simulink model "AssemControl"  (R2013a)
settings: Solver=ode15s  StartTime=0.0  StopTime=13  RelTol=1e-6
values from neighbouring files (symbols this model uses):
  Kd = [0.8784 0.9570 0.8952 0.9813 0.9602 1.0000]*koef*(-1)    [ParametriZaSimulacija.m]
  Ki = [0.1216 0.0430 0.1048 0.0187 0.0398 0]*koef    [ParametriZaSimulacija.m]
  Kp = [1.8784 1.9570 1.8952 1.9813 1.9602 2.0000]*koef*10    [ParametriZaSimulacija.m]
  q_pocetna = q_pocetna*pi/180    [ParametriZaSimulacija.m]
  s = size(xyz)    [PosakuvaniVremetraenja.m]    (also in invkine.m = size(theta_vl))
undefined symbols (not defined in the file or in its folder): X, Y, Z
libraries: sm_lib x450, fl_lib x46, nesl_utility x31
(part 5 of 9)

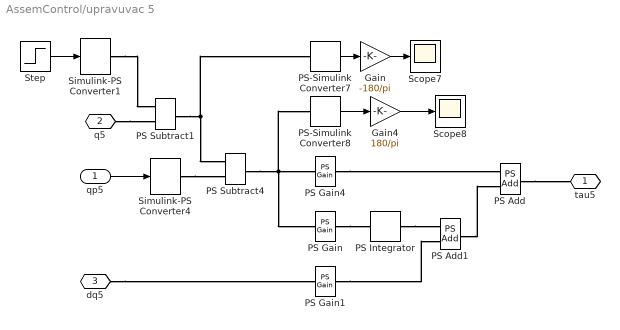
== system AssemControl/upravuvac 5 ==
  qp5 : Inport
  Gain : Gain  Gain=-180/pi
  Gain4 : Gain  Gain=180/pi
  PS Add : fl_lib/Physical Signals/Functions/PS Add  LocalVarLogging=[]
  PS Add1 : fl_lib/Physical Signals/Functions/PS Add  LocalVarLogging=[]
  PS Gain : fl_lib/Physical Signals/Functions/PS Gain  gain=Ki(5)  LocalVarLogging=[]
  PS Gain1 : fl_lib/Physical Signals/Functions/PS Gain  gain=Kd(5)  LocalVarLogging=[]
  PS Gain4 : fl_lib/Physical Signals/Functions/PS Gain  gain=Kp(5)  LocalVarLogging=[]
  PS Integrator : fl_lib/Physical Signals/Linear Operators/PS Integrator  x0=0  x_Log=off  LocalVarNames=|x  LocalVarDescs=|x  LocalVarLogging=0
  PS Subtract1 : fl_lib/Physical Signals/Functions/PS Subtract  LocalVarLogging=[]
  PS Subtract4 : fl_lib/Physical Signals/Functions/PS Subtract  LocalVarLogging=[]
  PS-Simulink Converter7 : nesl_utility/PS-Simulink Converter  PhysicalDomain=network_engine_domain  SubClassName=ps_output  LeftPortType=input  RightPortType=output  PseudoPeriodic=off  Frequencies=[]  Unit=1  AffineConversion=off
  PS-Simulink Converter8 : nesl_utility/PS-Simulink Converter  PhysicalDomain=network_engine_domain  SubClassName=ps_output  LeftPortType=input  RightPortType=output  PseudoPeriodic=off  Frequencies=[]  Unit=1  AffineConversion=off
  Scope7 : Scope
      settings: SaveName=ScopeData14
  Scope8 : Scope
      settings: SaveName=ScopeData3
  Simulink-PS Converter1 : nesl_utility/Simulink-PS Converter  PhysicalDomain=network_engine_domain  SubClassName=ps_input  LeftPortType=input  RightPortType=output  PseudoPeriodic=off  Frequencies=[]  NoiseDistribution=none  NoiseParameters=[]  Unit=1  AffineConversion=off  InputFiltering=off  SimscapeFilterOrder=1  InputFilterTimeConstant=0.001  UdotUserProvided=1
  Simulink-PS Converter4 : nesl_utility/Simulink-PS Converter  PhysicalDomain=network_engine_domain  SubClassName=ps_input  LeftPortType=input  RightPortType=output  PseudoPeriodic=off  Frequencies=[]  NoiseDistribution=none  NoiseParameters=[]  Unit=1  AffineConversion=off  InputFiltering=off  SimscapeFilterOrder=1  InputFilterTimeConstant=0.001  UdotUserProvided=1
  Step : Step  Time=0  Before=q_pocetna(5)  After=q_pocetna(5)  SampleTime=0
  tau5 : PMIOPort  Port=1  Side=Right
  q5 : PMIOPort  Port=2  Side=Left
  dq5 : PMIOPort  Port=3  Side=Left
  wires:
  qp5/1 -> Simulink-PS Converter4/1
  Step/1 -> Simulink-PS Converter1/1
  PS-Simulink Converter8/1 -> Gain4/1
  Gain4/1 -> Scope8/1
  PS-Simulink Converter7/1 -> Gain/1
  Gain/1 -> Scope7/1
  connections:
  PS Subtract1/RConn1 -- PS Subtract4/LConn2 -- PS-Simulink Converter7/LConn1
  PS Subtract4/RConn1 -- PS-Simulink Converter8/LConn1 -- PS Gain4/LConn1 -- PS Gain/LConn1
  Simulink-PS Converter4/RConn1 -- PS Subtract4/LConn1
  PS Add/RConn1 -- tau5/RConn1
  PS Gain4/RConn1 -- PS Add/LConn1
  PS Gain/RConn1 -- PS Integrator/LConn1
  PS Add1/RConn1 -- PS Add/LConn2
  PS Integrator/RConn1 -- PS Add1/LConn1
  PS Gain1/RConn1 -- PS Add1/LConn2
  dq5/RConn1 -- PS Gain1/LConn1
  Simulink-PS Converter1/RConn1 -- PS Subtract1/LConn2
  q5/RConn1 -- PS Subtract1/LConn1

== system AssemControl/upravuvac 6 ==
  qp6 : Inport
  Gain5 : Gain  Gain=-180/pi
  PS Gain5 : fl_lib/Physical Signals/Functions/PS Gain  gain=2000  LocalVarLogging=[]
  PS Subtract1 : fl_lib/Physical Signals/Functions/PS Subtract  LocalVarLogging=[]
  PS Subtract5 : fl_lib/Physical Signals/Functions/PS Subtract  LocalVarLogging=[]
  PS-Simulink Converter5 : nesl_utility/PS-Simulink Converter  PhysicalDomain=network_engine_domain  SubClassName=ps_output  LeftPortType=input  RightPortType=output  PseudoPeriodic=off  Frequencies=[]  Unit=1  AffineConversion=off
  Scope5 : Scope
      settings: YMin=-1.49252  YMax=-1.35038  SaveName=ScopeData11
  Simulink-PS Converter1 : nesl_utility/Simulink-PS Converter  PhysicalDomain=network_engine_domain  SubClassName=ps_input  LeftPortType=input  RightPortType=output  PseudoPeriodic=off  Frequencies=[]  NoiseDistribution=none  NoiseParameters=[]  Unit=1  AffineConversion=off  InputFiltering=off  SimscapeFilterOrder=1  InputFilterTimeConstant=0.001  UdotUserProvided=1
  Simulink-PS Converter5 : nesl_utility/Simulink-PS Converter  PhysicalDomain=network_engine_domain  SubClassName=ps_input  LeftPortType=input  RightPortType=output  PseudoPeriodic=off  Frequencies=[]  NoiseDistribution=none  NoiseParameters=[]  Unit=1  AffineConversion=off  InputFiltering=off  SimscapeFilterOrder=1  InputFilterTimeConstant=0.001  UdotUserProvided=1
  Step : Step  Time=0  Before=-0.2559  After=-0.2559  SampleTime=0
  tau6 : PMIOPort  Port=1  Side=Right
  q6 : PMIOPort  Port=2  Side=Left
  wires:
  PS-Simulink Converter5/1 -> Gain5/1
  Gain5/1 -> Scope5/1
  qp6/1 -> Simulink-PS Converter5/1
  Step/1 -> Simulink-PS Converter1/1
  connections:
  PS Subtract5/LConn2 -- PS Subtract1/RConn1 -- PS-Simulink Converter5/LConn1
  PS Subtract5/RConn1 -- PS Gain5/LConn1
  tau6/RConn1 -- PS Gain5/RConn1
  Simulink-PS Converter5/RConn1 -- PS Subtract5/LConn1
  Simulink-PS Converter1/RConn1 -- PS Subtract1/LConn2
  q6/RConn1 -- PS Subtract1/LConn1

== system AssemControl/Assem1_1_RIGID/Motor1_1_RIGID ==
  ReferenceFrame : sm_lib/Frames and  Transforms/Reference  Frame  BlockFunction=simmechanics.library.frames_transforms.reference_frame
  Solid : sm_lib/Body Elements/Solid  InertiaType=Custom  Mass=0.029311899999999998  MassUnits=kg  CenterOfMass=[0 -22.821300000000001 -9.8650699999999993]  CenterOfMassUnits=mm  MomentsOfInertia=[7.2099700000000002 5.1344899999999996 4.0333199999999998]  MomentsOfInertiaUnits=kg*mm^2  ProductsOfInertia=[0.19122700000000001 -4.5875100000000004e-09 0]  ProductsOfInertiaUnits=kg*mm^2  DensityBased=on  Density=1000  DensityUnits=kg/(m^3)  GraphicType=FromGeometry  MarkerShape=Sphere  MarkerSize=10  MarkerSizeUnits=m  GraphicVisPropType=SimpleVisualProperties  GraphicDiffuseColor=[0.25098 0.25098 0.25098]  GraphicSpecularColor=[0.5 0.5 0.5 1.0]  GraphicAmbientColor=[0.15 0.15 0.15 1.0]  GraphicEmissiveColor=[0.0 0.0 0.0 1.0]  GraphicShininess=75  GraphicOpacity=1  GeometryShape=FromFile  RectangleSize=[1 1]  RectangleSizeUnits=m  BrickDimensions=[1 1 1]  BrickDimensionUnits=m  CylinderRadius=1  CylinderRadiusUnits=m  CylinderLength=1  CylinderLengthUnits=m  SphereRadius=1  SphereRadiusUnits=m  EllipsoidRadii=[1 1 1]  EllipsoidRadiiUnits=m  ExtrusionCrossSection=[1 1; -1 1; -1 -1; 1 -1]  ExtrusionCrossSectionUnits=m  ExtrusionLength=1  ExtrusionLengthUnits=m  PolygonNumSides=3  PolygonOuterRadius=1  PolygonOuterRadiusUnits=m  ExtGeomFileName=Motor1_Default_sldprt.STL  ExtGeomFileUnits=mm  RevolutionCrossSection=[1 1; 1 -1; 2 -1; 2 1]  RevolutionCrossSectionUnits=m  RevolutionExtent=Full  RevolutionAngle=180  RevolutionAngleUnits=deg  BlockFunction=simmechanics.library.body_elements.solid
  F : PMIOPort  Port=1  Side=Left
  connections:
  Solid/RConn1 -- ReferenceFrame/RConn1 -- F/RConn1

== system AssemControl/Assem2_1_RIGID/Motor2_1_RIGID ==
  ReferenceFrame : sm_lib/Frames and  Transforms/Reference  Frame  BlockFunction=simmechanics.library.frames_transforms.reference_frame
  Solid : sm_lib/Body Elements/Solid  InertiaType=Custom  Mass=0.029311899999999998  MassUnits=kg  CenterOfMass=[0 -22.821300000000001 -9.8650699999999993]  CenterOfMassUnits=mm  MomentsOfInertia=[7.2099700000000002 5.1344899999999996 4.0333199999999998]  MomentsOfInertiaUnits=kg*mm^2  ProductsOfInertia=[0.19122700000000001 -4.5875100000000004e-09 0]  ProductsOfInertiaUnits=kg*mm^2  DensityBased=on  Density=1000  DensityUnits=kg/(m^3)  GraphicType=FromGeometry  MarkerShape=Sphere  MarkerSize=10  MarkerSizeUnits=m  GraphicVisPropType=SimpleVisualProperties  GraphicDiffuseColor=[0.25098 0.25098 0.25098]  GraphicSpecularColor=[0.5 0.5 0.5 1.0]  GraphicAmbientColor=[0.15 0.15 0.15 1.0]  GraphicEmissiveColor=[0.0 0.0 0.0 1.0]  GraphicShininess=75  GraphicOpacity=1  GeometryShape=FromFile  RectangleSize=[1 1]  RectangleSizeUnits=m  BrickDimensions=[1 1 1]  BrickDimensionUnits=m  CylinderRadius=1  CylinderRadiusUnits=m  CylinderLength=1  CylinderLengthUnits=m  SphereRadius=1  SphereRadiusUnits=m  EllipsoidRadii=[1 1 1]  EllipsoidRadiiUnits=m  ExtrusionCrossSection=[1 1; -1 1; -1 -1; 1 -1]  ExtrusionCrossSectionUnits=m  ExtrusionLength=1  ExtrusionLengthUnits=m  PolygonNumSides=3  PolygonOuterRadius=1  PolygonOuterRadiusUnits=m  ExtGeomFileName=Motor2_Default_sldprt.STL  ExtGeomFileUnits=mm  RevolutionCrossSection=[1 1; 1 -1; 2 -1; 2 1]  RevolutionCrossSectionUnits=m  RevolutionExtent=Full  RevolutionAngle=180  RevolutionAngleUnits=deg  BlockFunction=simmechanics.library.body_elements.solid
  F : PMIOPort  Port=1  Side=Left
  connections:
  Solid/RConn1 -- ReferenceFrame/RConn1 -- F/RConn1

== system AssemControl/Assem2_1_RIGID/Motor2_2_RIGID ==
  ReferenceFrame : sm_lib/Frames and  Transforms/Reference  Frame  BlockFunction=simmechanics.library.frames_transforms.reference_frame
  Solid : sm_lib/Body Elements/Solid  InertiaType=Custom  Mass=0.029311899999999998  MassUnits=kg  CenterOfMass=[0 -22.821300000000001 -9.8650699999999993]  CenterOfMassUnits=mm  MomentsOfInertia=[7.2099700000000002 5.1344899999999996 4.0333199999999998]  MomentsOfInertiaUnits=kg*mm^2  ProductsOfInertia=[0.19122700000000001 -4.5875100000000004e-09 0]  ProductsOfInertiaUnits=kg*mm^2  DensityBased=on  Density=1000  DensityUnits=kg/(m^3)  GraphicType=FromGeometry  MarkerShape=Sphere  MarkerSize=10  MarkerSizeUnits=m  GraphicVisPropType=SimpleVisualProperties  GraphicDiffuseColor=[0.25098 0.25098 0.25098]  GraphicSpecularColor=[0.5 0.5 0.5 1.0]  GraphicAmbientColor=[0.15 0.15 0.15 1.0]  GraphicEmissiveColor=[0.0 0.0 0.0 1.0]  GraphicShininess=75  GraphicOpacity=1  GeometryShape=FromFile  RectangleSize=[1 1]  RectangleSizeUnits=m  BrickDimensions=[1 1 1]  BrickDimensionUnits=m  CylinderRadius=1  CylinderRadiusUnits=m  CylinderLength=1  CylinderLengthUnits=m  SphereRadius=1  SphereRadiusUnits=m  EllipsoidRadii=[1 1 1]  EllipsoidRadiiUnits=m  ExtrusionCrossSection=[1 1; -1 1; -1 -1; 1 -1]  ExtrusionCrossSectionUnits=m  ExtrusionLength=1  ExtrusionLengthUnits=m  PolygonNumSides=3  PolygonOuterRadius=1  PolygonOuterRadiusUnits=m  ExtGeomFileName=Motor2_Default_sldprt.STL  ExtGeomFileUnits=mm  RevolutionCrossSection=[1 1; 1 -1; 2 -1; 2 1]  RevolutionCrossSectionUnits=m  RevolutionExtent=Full  RevolutionAngle=180  RevolutionAngleUnits=deg  BlockFunction=simmechanics.library.body_elements.solid
  F : PMIOPort  Port=1  Side=Left
  connections:
  Solid/RConn1 -- ReferenceFrame/RConn1 -- F/RConn1

== system AssemControl/Assem2_1_RIGID/Part1_1_RIGID ==
  ReferenceFrame : sm_lib/Frames and  Transforms/Reference  Frame  BlockFunction=simmechanics.library.frames_transforms.reference_frame
  Solid : sm_lib/Body Elements/Solid  InertiaType=Custom  Mass=0.061694100000000002  MassUnits=kg  CenterOfMass=[0 9.2105699999999988 -0.0014062]  CenterOfMassUnits=mm  MomentsOfInertia=[48.291799999999995 70.0852 51.645099999999999]  MomentsOfInertiaUnits=kg*mm^2  ProductsOfInertia=[-0.0020065700000000001 0 0]  ProductsOfInertiaUnits=kg*mm^2  DensityBased=on  Density=1000  DensityUnits=kg/(m^3)  GraphicType=FromGeometry  MarkerShape=Sphere  MarkerSize=10  MarkerSizeUnits=m  GraphicVisPropType=SimpleVisualProperties  GraphicDiffuseColor=[0.792157 0.819608 0.933333]  GraphicSpecularColor=[0.5 0.5 0.5 1.0]  GraphicAmbientColor=[0.15 0.15 0.15 1.0]  GraphicEmissiveColor=[0.0 0.0 0.0 1.0]  GraphicShininess=75  GraphicOpacity=1  GeometryShape=FromFile  RectangleSize=[1 1]  RectangleSizeUnits=m  BrickDimensions=[1 1 1]  BrickDimensionUnits=m  CylinderRadius=1  CylinderRadiusUnits=m  CylinderLength=1  CylinderLengthUnits=m  SphereRadius=1  SphereRadiusUnits=m  EllipsoidRadii=[1 1 1]  EllipsoidRadiiUnits=m  ExtrusionCrossSection=[1 1; -1 1; -1 -1; 1 -1]  ExtrusionCrossSectionUnits=m  ExtrusionLength=1  ExtrusionLengthUnits=m  PolygonNumSides=3  PolygonOuterRadius=1  PolygonOuterRadiusUnits=m  ExtGeomFileName=Part1_Default_sldprt.STL  ExtGeomFileUnits=mm  RevolutionCrossSection=[1 1; 1 -1; 2 -1; 2 1]  RevolutionCrossSectionUnits=m  RevolutionExtent=Full  RevolutionAngle=180  RevolutionAngleUnits=deg  BlockFunction=simmechanics.library.body_elements.solid
  F : PMIOPort  Port=1  Side=Left
  connections:
  Solid/RConn1 -- ReferenceFrame/RConn1 -- F/RConn1

== system AssemControl/Assem2_1_RIGID/navrtka1_1_RIGID ==
  ReferenceFrame : sm_lib/Frames and  Transforms/Reference  Frame  BlockFunction=simmechanics.library.frames_transforms.reference_frame
  Solid : sm_lib/Body Elements/Solid  InertiaType=Custom  Mass=4.2947000000000001e-05  MassUnits=kg  CenterOfMass=[0.000171375 -4.3854200000000001e-06 2.4601999999999998e-06]  CenterOfMassUnits=mm  MomentsOfInertia=[0.000130567 0.00013057200000000002 0.00019843399999999999]  MomentsOfInertiaUnits=kg*mm^2  ProductsOfInertia=[2.04154e-08 0 7.4980699999999995e-09]  ProductsOfInertiaUnits=kg*mm^2  DensityBased=on  Density=1000  DensityUnits=kg/(m^3)  GraphicType=FromGeometry  MarkerShape=Sphere  MarkerSize=10  MarkerSizeUnits=m  GraphicVisPropType=SimpleVisualProperties  GraphicDiffuseColor=[0.792157 0.819608 0.933333]  GraphicSpecularColor=[0.5 0.5 0.5 1.0]  GraphicAmbientColor=[0.15 0.15 0.15 1.0]  GraphicEmissiveColor=[0.0 0.0 0.0 1.0]  GraphicShininess=75  GraphicOpacity=1  GeometryShape=FromFile  RectangleSize=[1 1]  RectangleSizeUnits=m  BrickDimensions=[1 1 1]  BrickDimensionUnits=m  CylinderRadius=1  CylinderRadiusUnits=m  CylinderLength=1  CylinderLengthUnits=m  SphereRadius=1  SphereRadiusUnits=m  EllipsoidRadii=[1 1 1]  EllipsoidRadiiUnits=m  ExtrusionCrossSection=[1 1; -1 1; -1 -1; 1 -1]  ExtrusionCrossSectionUnits=m  ExtrusionLength=1  ExtrusionLengthUnits=m  PolygonNumSides=3  PolygonOuterRadius=1  PolygonOuterRadiusUnits=m  ExtGeomFileName=navrtka1_Default_sldprt.STL  ExtGeomFileUnits=mm  RevolutionCrossSection=[1 1; 1 -1; 2 -1; 2 1]  RevolutionCrossSectionUnits=m  RevolutionExtent=Full  RevolutionAngle=180  RevolutionAngleUnits=deg  BlockFunction=simmechanics.library.body_elements.solid
  F : PMIOPort  Port=1  Side=Left
  connections:
  Solid/RConn1 -- ReferenceFrame/RConn1 -- F/RConn1

== system AssemControl/Assem2_1_RIGID/navrtka1_2_RIGID ==
  ReferenceFrame : sm_lib/Frames and  Transforms/Reference  Frame  BlockFunction=simmechanics.library.frames_transforms.reference_frame
  Solid : sm_lib/Body Elements/Solid  InertiaType=Custom  Mass=4.2947000000000001e-05  MassUnits=kg  CenterOfMass=[0.000171375 -4.3854200000000001e-06 2.4601999999999998e-06]  CenterOfMassUnits=mm  MomentsOfInertia=[0.000130567 0.00013057200000000002 0.00019843399999999999]  MomentsOfInertiaUnits=kg*mm^2  ProductsOfInertia=[2.04154e-08 0 7.4980699999999995e-09]  ProductsOfInertiaUnits=kg*mm^2  DensityBased=on  Density=1000  DensityUnits=kg/(m^3)  GraphicType=FromGeometry  MarkerShape=Sphere  MarkerSize=10  MarkerSizeUnits=m  GraphicVisPropType=SimpleVisualProperties  GraphicDiffuseColor=[0.792157 0.819608 0.933333]  GraphicSpecularColor=[0.5 0.5 0.5 1.0]  GraphicAmbientColor=[0.15 0.15 0.15 1.0]  GraphicEmissiveColor=[0.0 0.0 0.0 1.0]  GraphicShininess=75  GraphicOpacity=1  GeometryShape=FromFile  RectangleSize=[1 1]  RectangleSizeUnits=m  BrickDimensions=[1 1 1]  BrickDimensionUnits=m  CylinderRadius=1  CylinderRadiusUnits=m  CylinderLength=1  CylinderLengthUnits=m  SphereRadius=1  SphereRadiusUnits=m  EllipsoidRadii=[1 1 1]  EllipsoidRadiiUnits=m  ExtrusionCrossSection=[1 1; -1 1; -1 -1; 1 -1]  ExtrusionCrossSectionUnits=m  ExtrusionLength=1  ExtrusionLengthUnits=m  PolygonNumSides=3  PolygonOuterRadius=1  PolygonOuterRadiusUnits=m  ExtGeomFileName=navrtka1_Default_sldprt.STL  ExtGeomFileUnits=mm  RevolutionCrossSection=[1 1; 1 -1; 2 -1; 2 1]  RevolutionCrossSectionUnits=m  RevolutionExtent=Full  RevolutionAngle=180  RevolutionAngleUnits=deg  BlockFunction=simmechanics.library.body_elements.solid
  F : PMIOPort  Port=1  Side=Left
  connections:
  Solid/RConn1 -- ReferenceFrame/RConn1 -- F/RConn1

== system AssemControl/Assem2_1_RIGID/navrtka1_3_RIGID ==
  ReferenceFrame : sm_lib/Frames and  Transforms/Reference  Frame  BlockFunction=simmechanics.library.frames_transforms.reference_frame
  Solid : sm_lib/Body Elements/Solid  InertiaType=Custom  Mass=4.2947000000000001e-05  MassUnits=kg  CenterOfMass=[0.000171375 -4.3854200000000001e-06 2.4601999999999998e-06]  CenterOfMassUnits=mm  MomentsOfInertia=[0.000130567 0.00013057200000000002 0.00019843399999999999]  MomentsOfInertiaUnits=kg*mm^2  ProductsOfInertia=[2.04154e-08 0 7.4980699999999995e-09]  ProductsOfInertiaUnits=kg*mm^2  DensityBased=on  Density=1000  DensityUnits=kg/(m^3)  GraphicType=FromGeometry  MarkerShape=Sphere  MarkerSize=10  MarkerSizeUnits=m  GraphicVisPropType=SimpleVisualProperties  GraphicDiffuseColor=[0.792157 0.819608 0.933333]  GraphicSpecularColor=[0.5 0.5 0.5 1.0]  GraphicAmbientColor=[0.15 0.15 0.15 1.0]  GraphicEmissiveColor=[0.0 0.0 0.0 1.0]  GraphicShininess=75  GraphicOpacity=1  GeometryShape=FromFile  RectangleSize=[1 1]  RectangleSizeUnits=m  BrickDimensions=[1 1 1]  BrickDimensionUnits=m  CylinderRadius=1  CylinderRadiusUnits=m  CylinderLength=1  CylinderLengthUnits=m  SphereRadius=1  SphereRadiusUnits=m  EllipsoidRadii=[1 1 1]  EllipsoidRadiiUnits=m  ExtrusionCrossSection=[1 1; -1 1; -1 -1; 1 -1]  ExtrusionCrossSectionUnits=m  ExtrusionLength=1  ExtrusionLengthUnits=m  PolygonNumSides=3  PolygonOuterRadius=1  PolygonOuterRadiusUnits=m  ExtGeomFileName=navrtka1_Default_sldprt.STL  ExtGeomFileUnits=mm  RevolutionCrossSection=[1 1; 1 -1; 2 -1; 2 1]  RevolutionCrossSectionUnits=m  RevolutionExtent=Full  RevolutionAngle=180  RevolutionAngleUnits=deg  BlockFunction=simmechanics.library.body_elements.solid
  F : PMIOPort  Port=1  Side=Left
  connections:
  Solid/RConn1 -- ReferenceFrame/RConn1 -- F/RConn1

== system AssemControl/Assem2_1_RIGID/navrtka1_4_RIGID ==
  ReferenceFrame : sm_lib/Frames and  Transforms/Reference  Frame  BlockFunction=simmechanics.library.frames_transforms.reference_frame
  Solid : sm_lib/Body Elements/Solid  InertiaType=Custom  Mass=4.2947000000000001e-05  MassUnits=kg  CenterOfMass=[0.000171375 -4.3854200000000001e-06 2.4601999999999998e-06]  CenterOfMassUnits=mm  MomentsOfInertia=[0.000130567 0.00013057200000000002 0.00019843399999999999]  MomentsOfInertiaUnits=kg*mm^2  ProductsOfInertia=[2.04154e-08 0 7.4980699999999995e-09]  ProductsOfInertiaUnits=kg*mm^2  DensityBased=on  Density=1000  DensityUnits=kg/(m^3)  GraphicType=FromGeometry  MarkerShape=Sphere  MarkerSize=10  MarkerSizeUnits=m  GraphicVisPropType=SimpleVisualProperties  GraphicDiffuseColor=[0.792157 0.819608 0.933333]  GraphicSpecularColor=[0.5 0.5 0.5 1.0]  GraphicAmbientColor=[0.15 0.15 0.15 1.0]  GraphicEmissiveColor=[0.0 0.0 0.0 1.0]  GraphicShininess=75  GraphicOpacity=1  GeometryShape=FromFile  RectangleSize=[1 1]  RectangleSizeUnits=m  BrickDimensions=[1 1 1]  BrickDimensionUnits=m  CylinderRadius=1  CylinderRadiusUnits=m  CylinderLength=1  CylinderLengthUnits=m  SphereRadius=1  SphereRadiusUnits=m  EllipsoidRadii=[1 1 1]  EllipsoidRadiiUnits=m  ExtrusionCrossSection=[1 1; -1 1; -1 -1; 1 -1]  ExtrusionCrossSectionUnits=m  ExtrusionLength=1  ExtrusionLengthUnits=m  PolygonNumSides=3  PolygonOuterRadius=1  PolygonOuterRadiusUnits=m  ExtGeomFileName=navrtka1_Default_sldprt.STL  ExtGeomFileUnits=mm  RevolutionCrossSection=[1 1; 1 -1; 2 -1; 2 1]  RevolutionCrossSectionUnits=m  RevolutionExtent=Full  RevolutionAngle=180  RevolutionAngleUnits=deg  BlockFunction=simmechanics.library.body_elements.solid
  F : PMIOPort  Port=1  Side=Left
  connections:
  Solid/RConn1 -- ReferenceFrame/RConn1 -- F/RConn1

== system AssemControl/Assem2_1_RIGID/navrtka1_5_RIGID ==
  ReferenceFrame : sm_lib/Frames and  Transforms/Reference  Frame  BlockFunction=simmechanics.library.frames_transforms.reference_frame
  Solid : sm_lib/Body Elements/Solid  InertiaType=Custom  Mass=4.2947000000000001e-05  MassUnits=kg  CenterOfMass=[0.000171375 -4.3854200000000001e-06 2.4601999999999998e-06]  CenterOfMassUnits=mm  MomentsOfInertia=[0.000130567 0.00013057200000000002 0.00019843399999999999]  MomentsOfInertiaUnits=kg*mm^2  ProductsOfInertia=[2.04154e-08 0 7.4980699999999995e-09]  ProductsOfInertiaUnits=kg*mm^2  DensityBased=on  Density=1000  DensityUnits=kg/(m^3)  GraphicType=FromGeometry  MarkerShape=Sphere  MarkerSize=10  MarkerSizeUnits=m  GraphicVisPropType=SimpleVisualProperties  GraphicDiffuseColor=[0.792157 0.819608 0.933333]  GraphicSpecularColor=[0.5 0.5 0.5 1.0]  GraphicAmbientColor=[0.15 0.15 0.15 1.0]  GraphicEmissiveColor=[0.0 0.0 0.0 1.0]  GraphicShininess=75  GraphicOpacity=1  GeometryShape=FromFile  RectangleSize=[1 1]  RectangleSizeUnits=m  BrickDimensions=[1 1 1]  BrickDimensionUnits=m  CylinderRadius=1  CylinderRadiusUnits=m  CylinderLength=1  CylinderLengthUnits=m  SphereRadius=1  SphereRadiusUnits=m  EllipsoidRadii=[1 1 1]  EllipsoidRadiiUnits=m  ExtrusionCrossSection=[1 1; -1 1; -1 -1; 1 -1]  ExtrusionCrossSectionUnits=m  ExtrusionLength=1  ExtrusionLengthUnits=m  PolygonNumSides=3  PolygonOuterRadius=1  PolygonOuterRadiusUnits=m  ExtGeomFileName=navrtka1_Default_sldprt.STL  ExtGeomFileUnits=mm  RevolutionCrossSection=[1 1; 1 -1; 2 -1; 2 1]  RevolutionCrossSectionUnits=m  RevolutionExtent=Full  RevolutionAngle=180  RevolutionAngleUnits=deg  BlockFunction=simmechanics.library.body_elements.solid
  F : PMIOPort  Port=1  Side=Left
  connections:
  Solid/RConn1 -- ReferenceFrame/RConn1 -- F/RConn1

== system AssemControl/Assem2_1_RIGID/navrtka1_6_RIGID ==
  ReferenceFrame : sm_lib/Frames and  Transforms/Reference  Frame  BlockFunction=simmechanics.library.frames_transforms.reference_frame
  Solid : sm_lib/Body Elements/Solid  InertiaType=Custom  Mass=4.2947000000000001e-05  MassUnits=kg  CenterOfMass=[0.000171375 -4.3854200000000001e-06 2.4601999999999998e-06]  CenterOfMassUnits=mm  MomentsOfInertia=[0.000130567 0.00013057200000000002 0.00019843399999999999]  MomentsOfInertiaUnits=kg*mm^2  ProductsOfInertia=[2.04154e-08 0 7.4980699999999995e-09]  ProductsOfInertiaUnits=kg*mm^2  DensityBased=on  Density=1000  DensityUnits=kg/(m^3)  GraphicType=FromGeometry  MarkerShape=Sphere  MarkerSize=10  MarkerSizeUnits=m  GraphicVisPropType=SimpleVisualProperties  GraphicDiffuseColor=[0.792157 0.819608 0.933333]  GraphicSpecularColor=[0.5 0.5 0.5 1.0]  GraphicAmbientColor=[0.15 0.15 0.15 1.0]  GraphicEmissiveColor=[0.0 0.0 0.0 1.0]  GraphicShininess=75  GraphicOpacity=1  GeometryShape=FromFile  RectangleSize=[1 1]  RectangleSizeUnits=m  BrickDimensions=[1 1 1]  BrickDimensionUnits=m  CylinderRadius=1  CylinderRadiusUnits=m  CylinderLength=1  CylinderLengthUnits=m  SphereRadius=1  SphereRadiusUnits=m  EllipsoidRadii=[1 1 1]  EllipsoidRadiiUnits=m  ExtrusionCrossSection=[1 1; -1 1; -1 -1; 1 -1]  ExtrusionCrossSectionUnits=m  ExtrusionLength=1  ExtrusionLengthUnits=m  PolygonNumSides=3  PolygonOuterRadius=1  PolygonOuterRadiusUnits=m  ExtGeomFileName=navrtka1_Default_sldprt.STL  ExtGeomFileUnits=mm  RevolutionCrossSection=[1 1; 1 -1; 2 -1; 2 1]  RevolutionCrossSectionUnits=m  RevolutionExtent=Full  RevolutionAngle=180  RevolutionAngleUnits=deg  BlockFunction=simmechanics.library.body_elements.solid
  F : PMIOPort  Port=1  Side=Left
  connections:
  Solid/RConn1 -- ReferenceFrame/RConn1 -- F/RConn1

== system AssemControl/Assem2_1_RIGID/navrtka1_7_RIGID ==
  ReferenceFrame : sm_lib/Frames and  Transforms/Reference  Frame  BlockFunction=simmechanics.library.frames_transforms.reference_frame
  Solid : sm_lib/Body Elements/Solid  InertiaType=Custom  Mass=4.2947000000000001e-05  MassUnits=kg  CenterOfMass=[0.000171375 -4.3854200000000001e-06 2.4601999999999998e-06]  CenterOfMassUnits=mm  MomentsOfInertia=[0.000130567 0.00013057200000000002 0.00019843399999999999]  MomentsOfInertiaUnits=kg*mm^2  ProductsOfInertia=[2.04154e-08 0 7.4980699999999995e-09]  ProductsOfInertiaUnits=kg*mm^2  DensityBased=on  Density=1000  DensityUnits=kg/(m^3)  GraphicType=FromGeometry  MarkerShape=Sphere  MarkerSize=10  MarkerSizeUnits=m  GraphicVisPropType=SimpleVisualProperties  GraphicDiffuseColor=[0.792157 0.819608 0.933333]  GraphicSpecularColor=[0.5 0.5 0.5 1.0]  GraphicAmbientColor=[0.15 0.15 0.15 1.0]  GraphicEmissiveColor=[0.0 0.0 0.0 1.0]  GraphicShininess=75  GraphicOpacity=1  GeometryShape=FromFile  RectangleSize=[1 1]  RectangleSizeUnits=m  BrickDimensions=[1 1 1]  BrickDimensionUnits=m  CylinderRadius=1  CylinderRadiusUnits=m  CylinderLength=1  CylinderLengthUnits=m  SphereRadius=1  SphereRadiusUnits=m  EllipsoidRadii=[1 1 1]  EllipsoidRadiiUnits=m  ExtrusionCrossSection=[1 1; -1 1; -1 -1; 1 -1]  ExtrusionCrossSectionUnits=m  ExtrusionLength=1  ExtrusionLengthUnits=m  PolygonNumSides=3  PolygonOuterRadius=1  PolygonOuterRadiusUnits=m  ExtGeomFileName=navrtka1_Default_sldprt.STL  ExtGeomFileUnits=mm  RevolutionCrossSection=[1 1; 1 -1; 2 -1; 2 1]  RevolutionCrossSectionUnits=m  RevolutionExtent=Full  RevolutionAngle=180  RevolutionAngleUnits=deg  BlockFunction=simmechanics.library.body_elements.solid
  F : PMIOPort  Port=1  Side=Left
  connections:
  Solid/RConn1 -- ReferenceFrame/RConn1 -- F/RConn1

== system AssemControl/Assem2_1_RIGID/navrtka1_8_RIGID ==
  ReferenceFrame : sm_lib/Frames and  Transforms/Reference  Frame  BlockFunction=simmechanics.library.frames_transforms.reference_frame
  Solid : sm_lib/Body Elements/Solid  InertiaType=Custom  Mass=4.2947000000000001e-05  MassUnits=kg  CenterOfMass=[0.000171375 -4.3854200000000001e-06 2.4601999999999998e-06]  CenterOfMassUnits=mm  MomentsOfInertia=[0.000130567 0.00013057200000000002 0.00019843399999999999]  MomentsOfInertiaUnits=kg*mm^2  ProductsOfInertia=[2.04154e-08 0 7.4980699999999995e-09]  ProductsOfInertiaUnits=kg*mm^2  DensityBased=on  Density=1000  DensityUnits=kg/(m^3)  GraphicType=FromGeometry  MarkerShape=Sphere  MarkerSize=10  MarkerSizeUnits=m  GraphicVisPropType=SimpleVisualProperties  GraphicDiffuseColor=[0.792157 0.819608 0.933333]  GraphicSpecularColor=[0.5 0.5 0.5 1.0]  GraphicAmbientColor=[0.15 0.15 0.15 1.0]  GraphicEmissiveColor=[0.0 0.0 0.0 1.0]  GraphicShininess=75  GraphicOpacity=1  GeometryShape=FromFile  RectangleSize=[1 1]  RectangleSizeUnits=m  BrickDimensions=[1 1 1]  BrickDimensionUnits=m  CylinderRadius=1  CylinderRadiusUnits=m  CylinderLength=1  CylinderLengthUnits=m  SphereRadius=1  SphereRadiusUnits=m  EllipsoidRadii=[1 1 1]  EllipsoidRadiiUnits=m  ExtrusionCrossSection=[1 1; -1 1; -1 -1; 1 -1]  ExtrusionCrossSectionUnits=m  ExtrusionLength=1  ExtrusionLengthUnits=m  PolygonNumSides=3  PolygonOuterRadius=1  PolygonOuterRadiusUnits=m  ExtGeomFileName=navrtka1_Default_sldprt.STL  ExtGeomFileUnits=mm  RevolutionCrossSection=[1 1; 1 -1; 2 -1; 2 1]  RevolutionCrossSectionUnits=m  RevolutionExtent=Full  RevolutionAngle=180  RevolutionAngleUnits=deg  BlockFunction=simmechanics.library.body_elements.solid
  F : PMIOPort  Port=1  Side=Left
  connections:
  Solid/RConn1 -- ReferenceFrame/RConn1 -- F/RConn1

== system AssemControl/Assem2_1_RIGID/straf3_dolg11_1_RIGID ==
  ReferenceFrame : sm_lib/Frames and  Transforms/Reference  Frame  BlockFunction=simmechanics.library.frames_transforms.reference_frame
  Solid : sm_lib/Body Elements/Solid  InertiaType=Custom  Mass=0.000114876  MassUnits=kg  CenterOfMass=[-1.42702 -0.0032510100000000004 0.00051650799999999994]  CenterOfMassUnits=mm  MomentsOfInertia=[0.00026421799999999998 0.0019891899999999996 0.0019891700000000002]  MomentsOfInertiaUnits=kg*mm^2  ProductsOfInertia=[-1.31544e-07 -5.9438499999999999e-07 -2.3482500000000001e-07]  ProductsOfInertiaUnits=kg*mm^2  DensityBased=on  Density=1000  DensityUnits=kg/(m^3)  GraphicType=FromGeometry  MarkerShape=Sphere  MarkerSize=10  MarkerSizeUnits=m  GraphicVisPropType=SimpleVisualProperties  GraphicDiffuseColor=[0.792157 0.819608 0.933333]  GraphicSpecularColor=[0.5 0.5 0.5 1.0]  GraphicAmbientColor=[0.15 0.15 0.15 1.0]  GraphicEmissiveColor=[0.0 0.0 0.0 1.0]  GraphicShininess=75  GraphicOpacity=1  GeometryShape=FromFile  RectangleSize=[1 1]  RectangleSizeUnits=m  BrickDimensions=[1 1 1]  BrickDimensionUnits=m  CylinderRadius=1  CylinderRadiusUnits=m  CylinderLength=1  CylinderLengthUnits=m  SphereRadius=1  SphereRadiusUnits=m  EllipsoidRadii=[1 1 1]  EllipsoidRadiiUnits=m  ExtrusionCrossSection=[1 1; -1 1; -1 -1; 1 -1]  ExtrusionCrossSectionUnits=m  ExtrusionLength=1  ExtrusionLengthUnits=m  PolygonNumSides=3  PolygonOuterRadius=1  PolygonOuterRadiusUnits=m  ExtGeomFileName=straf3_dolg11_Default_sldprt.STL  ExtGeomFileUnits=mm  RevolutionCrossSection=[1 1; 1 -1; 2 -1; 2 1]  RevolutionCrossSectionUnits=m  RevolutionExtent=Full  RevolutionAngle=180  RevolutionAngleUnits=deg  BlockFunction=simmechanics.library.body_elements.solid
  F : PMIOPort  Port=1  Side=Left
  connections:
  Solid/RConn1 -- ReferenceFrame/RConn1 -- F/RConn1

== system AssemControl/Assem2_1_RIGID/straf3_dolg11_2_RIGID ==
  ReferenceFrame : sm_lib/Frames and  Transforms/Reference  Frame  BlockFunction=simmechanics.library.frames_transforms.reference_frame
  Solid : sm_lib/Body Elements/Solid  InertiaType=Custom  Mass=0.000114876  MassUnits=kg  CenterOfMass=[-1.42702 -0.0032510100000000004 0.00051650799999999994]  CenterOfMassUnits=mm  MomentsOfInertia=[0.00026421799999999998 0.0019891899999999996 0.0019891700000000002]  MomentsOfInertiaUnits=kg*mm^2  ProductsOfInertia=[-1.31544e-07 -5.9438499999999999e-07 -2.3482500000000001e-07]  ProductsOfInertiaUnits=kg*mm^2  DensityBased=on  Density=1000  DensityUnits=kg/(m^3)  GraphicType=FromGeometry  MarkerShape=Sphere  MarkerSize=10  MarkerSizeUnits=m  GraphicVisPropType=SimpleVisualProperties  GraphicDiffuseColor=[0.792157 0.819608 0.933333]  GraphicSpecularColor=[0.5 0.5 0.5 1.0]  GraphicAmbientColor=[0.15 0.15 0.15 1.0]  GraphicEmissiveColor=[0.0 0.0 0.0 1.0]  GraphicShininess=75  GraphicOpacity=1  GeometryShape=FromFile  RectangleSize=[1 1]  RectangleSizeUnits=m  BrickDimensions=[1 1 1]  BrickDimensionUnits=m  CylinderRadius=1  CylinderRadiusUnits=m  CylinderLength=1  CylinderLengthUnits=m  SphereRadius=1  SphereRadiusUnits=m  EllipsoidRadii=[1 1 1]  EllipsoidRadiiUnits=m  ExtrusionCrossSection=[1 1; -1 1; -1 -1; 1 -1]  ExtrusionCrossSectionUnits=m  ExtrusionLength=1  ExtrusionLengthUnits=m  PolygonNumSides=3  PolygonOuterRadius=1  PolygonOuterRadiusUnits=m  ExtGeomFileName=straf3_dolg11_Default_sldprt.STL  ExtGeomFileUnits=mm  RevolutionCrossSection=[1 1; 1 -1; 2 -1; 2 1]  RevolutionCrossSectionUnits=m  RevolutionExtent=Full  RevolutionAngle=180  RevolutionAngleUnits=deg  BlockFunction=simmechanics.library.body_elements.solid
  F : PMIOPort  Port=1  Side=Left
  connections:
  Solid/RConn1 -- ReferenceFrame/RConn1 -- F/RConn1

== system AssemControl/Assem2_1_RIGID/straf3_dolg11_3_RIGID ==
  ReferenceFrame : sm_lib/Frames and  Transforms/Reference  Frame  BlockFunction=simmechanics.library.frames_transforms.reference_frame
  Solid : sm_lib/Body Elements/Solid  InertiaType=Custom  Mass=0.000114876  MassUnits=kg  CenterOfMass=[-1.42702 -0.0032510100000000004 0.00051650799999999994]  CenterOfMassUnits=mm  MomentsOfInertia=[0.00026421799999999998 0.0019891899999999996 0.0019891700000000002]  MomentsOfInertiaUnits=kg*mm^2  ProductsOfInertia=[-1.31544e-07 -5.9438499999999999e-07 -2.3482500000000001e-07]  ProductsOfInertiaUnits=kg*mm^2  DensityBased=on  Density=1000  DensityUnits=kg/(m^3)  GraphicType=FromGeometry  MarkerShape=Sphere  MarkerSize=10  MarkerSizeUnits=m  GraphicVisPropType=SimpleVisualProperties  GraphicDiffuseColor=[0.792157 0.819608 0.933333]  GraphicSpecularColor=[0.5 0.5 0.5 1.0]  GraphicAmbientColor=[0.15 0.15 0.15 1.0]  GraphicEmissiveColor=[0.0 0.0 0.0 1.0]  GraphicShininess=75  GraphicOpacity=1  GeometryShape=FromFile  RectangleSize=[1 1]  RectangleSizeUnits=m  BrickDimensions=[1 1 1]  BrickDimensionUnits=m  CylinderRadius=1  CylinderRadiusUnits=m  CylinderLength=1  CylinderLengthUnits=m  SphereRadius=1  SphereRadiusUnits=m  EllipsoidRadii=[1 1 1]  EllipsoidRadiiUnits=m  ExtrusionCrossSection=[1 1; -1 1; -1 -1; 1 -1]  ExtrusionCrossSectionUnits=m  ExtrusionLength=1  ExtrusionLengthUnits=m  PolygonNumSides=3  PolygonOuterRadius=1  PolygonOuterRadiusUnits=m  ExtGeomFileName=straf3_dolg11_Default_sldprt.STL  ExtGeomFileUnits=mm  RevolutionCrossSection=[1 1; 1 -1; 2 -1; 2 1]  RevolutionCrossSectionUnits=m  RevolutionExtent=Full  RevolutionAngle=180  RevolutionAngleUnits=deg  BlockFunction=simmechanics.library.body_elements.solid
  F : PMIOPort  Port=1  Side=Left
  connections:
  Solid/RConn1 -- ReferenceFrame/RConn1 -- F/RConn1

== system AssemControl/Assem2_1_RIGID/straf3_dolg11_4_RIGID ==
  ReferenceFrame : sm_lib/Frames and  Transforms/Reference  Frame  BlockFunction=simmechanics.library.frames_transforms.reference_frame
  Solid : sm_lib/Body Elements/Solid  InertiaType=Custom  Mass=0.000114876  MassUnits=kg  CenterOfMass=[-1.42702 -0.0032510100000000004 0.00051650799999999994]  CenterOfMassUnits=mm  MomentsOfInertia=[0.00026421799999999998 0.0019891899999999996 0.0019891700000000002]  MomentsOfInertiaUnits=kg*mm^2  ProductsOfInertia=[-1.31544e-07 -5.9438499999999999e-07 -2.3482500000000001e-07]  ProductsOfInertiaUnits=kg*mm^2  DensityBased=on  Density=1000  DensityUnits=kg/(m^3)  GraphicType=FromGeometry  MarkerShape=Sphere  MarkerSize=10  MarkerSizeUnits=m  GraphicVisPropType=SimpleVisualProperties  GraphicDiffuseColor=[0.792157 0.819608 0.933333]  GraphicSpecularColor=[0.5 0.5 0.5 1.0]  GraphicAmbientColor=[0.15 0.15 0.15 1.0]  GraphicEmissiveColor=[0.0 0.0 0.0 1.0]  GraphicShininess=75  GraphicOpacity=1  GeometryShape=FromFile  RectangleSize=[1 1]  RectangleSizeUnits=m  BrickDimensions=[1 1 1]  BrickDimensionUnits=m  CylinderRadius=1  CylinderRadiusUnits=m  CylinderLength=1  CylinderLengthUnits=m  SphereRadius=1  SphereRadiusUnits=m  EllipsoidRadii=[1 1 1]  EllipsoidRadiiUnits=m  ExtrusionCrossSection=[1 1; -1 1; -1 -1; 1 -1]  ExtrusionCrossSectionUnits=m  ExtrusionLength=1  ExtrusionLengthUnits=m  PolygonNumSides=3  PolygonOuterRadius=1  PolygonOuterRadiusUnits=m  ExtGeomFileName=straf3_dolg11_Default_sldprt.STL  ExtGeomFileUnits=mm  RevolutionCrossSection=[1 1; 1 -1; 2 -1; 2 1]  RevolutionCrossSectionUnits=m  RevolutionExtent=Full  RevolutionAngle=180  RevolutionAngleUnits=deg  BlockFunction=simmechanics.library.body_elements.solid
  F : PMIOPort  Port=1  Side=Left
  connections:
  Solid/RConn1 -- ReferenceFrame/RConn1 -- F/RConn1

== system AssemControl/Assem2_1_RIGID/straf3_dolg11_5_RIGID ==
  ReferenceFrame : sm_lib/Frames and  Transforms/Reference  Frame  BlockFunction=simmechanics.library.frames_transforms.reference_frame
  Solid : sm_lib/Body Elements/Solid  InertiaType=Custom  Mass=0.000114876  MassUnits=kg  CenterOfMass=[-1.42702 -0.0032510100000000004 0.00051650799999999994]  CenterOfMassUnits=mm  MomentsOfInertia=[0.00026421799999999998 0.0019891899999999996 0.0019891700000000002]  MomentsOfInertiaUnits=kg*mm^2  ProductsOfInertia=[-1.31544e-07 -5.9438499999999999e-07 -2.3482500000000001e-07]  ProductsOfInertiaUnits=kg*mm^2  DensityBased=on  Density=1000  DensityUnits=kg/(m^3)  GraphicType=FromGeometry  MarkerShape=Sphere  MarkerSize=10  MarkerSizeUnits=m  GraphicVisPropType=SimpleVisualProperties  GraphicDiffuseColor=[0.792157 0.819608 0.933333]  GraphicSpecularColor=[0.5 0.5 0.5 1.0]  GraphicAmbientColor=[0.15 0.15 0.15 1.0]  GraphicEmissiveColor=[0.0 0.0 0.0 1.0]  GraphicShininess=75  GraphicOpacity=1  GeometryShape=FromFile  RectangleSize=[1 1]  RectangleSizeUnits=m  BrickDimensions=[1 1 1]  BrickDimensionUnits=m  CylinderRadius=1  CylinderRadiusUnits=m  CylinderLength=1  CylinderLengthUnits=m  SphereRadius=1  SphereRadiusUnits=m  EllipsoidRadii=[1 1 1]  EllipsoidRadiiUnits=m  ExtrusionCrossSection=[1 1; -1 1; -1 -1; 1 -1]  ExtrusionCrossSectionUnits=m  ExtrusionLength=1  ExtrusionLengthUnits=m  PolygonNumSides=3  PolygonOuterRadius=1  PolygonOuterRadiusUnits=m  ExtGeomFileName=straf3_dolg11_Default_sldprt.STL  ExtGeomFileUnits=mm  RevolutionCrossSection=[1 1; 1 -1; 2 -1; 2 1]  RevolutionCrossSectionUnits=m  RevolutionExtent=Full  RevolutionAngle=180  RevolutionAngleUnits=deg  BlockFunction=simmechanics.library.body_elements.solid
  F : PMIOPort  Port=1  Side=Left
  connections:
  Solid/RConn1 -- ReferenceFrame/RConn1 -- F/RConn1

== system AssemControl/Assem2_1_RIGID/straf3_dolg11_6_RIGID ==
  ReferenceFrame : sm_lib/Frames and  Transforms/Reference  Frame  BlockFunction=simmechanics.library.frames_transforms.reference_frame
  Solid : sm_lib/Body Elements/Solid  InertiaType=Custom  Mass=0.000114876  MassUnits=kg  CenterOfMass=[-1.42702 -0.0032510100000000004 0.00051650799999999994]  CenterOfMassUnits=mm  MomentsOfInertia=[0.00026421799999999998 0.0019891899999999996 0.0019891700000000002]  MomentsOfInertiaUnits=kg*mm^2  ProductsOfInertia=[-1.31544e-07 -5.9438499999999999e-07 -2.3482500000000001e-07]  ProductsOfInertiaUnits=kg*mm^2  DensityBased=on  Density=1000  DensityUnits=kg/(m^3)  GraphicType=FromGeometry  MarkerShape=Sphere  MarkerSize=10  MarkerSizeUnits=m  GraphicVisPropType=SimpleVisualProperties  GraphicDiffuseColor=[0.792157 0.819608 0.933333]  GraphicSpecularColor=[0.5 0.5 0.5 1.0]  GraphicAmbientColor=[0.15 0.15 0.15 1.0]  GraphicEmissiveColor=[0.0 0.0 0.0 1.0]  GraphicShininess=75  GraphicOpacity=1  GeometryShape=FromFile  RectangleSize=[1 1]  RectangleSizeUnits=m  BrickDimensions=[1 1 1]  BrickDimensionUnits=m  CylinderRadius=1  CylinderRadiusUnits=m  CylinderLength=1  CylinderLengthUnits=m  SphereRadius=1  SphereRadiusUnits=m  EllipsoidRadii=[1 1 1]  EllipsoidRadiiUnits=m  ExtrusionCrossSection=[1 1; -1 1; -1 -1; 1 -1]  ExtrusionCrossSectionUnits=m  ExtrusionLength=1  ExtrusionLengthUnits=m  PolygonNumSides=3  PolygonOuterRadius=1  PolygonOuterRadiusUnits=m  ExtGeomFileName=straf3_dolg11_Default_sldprt.STL  ExtGeomFileUnits=mm  RevolutionCrossSection=[1 1; 1 -1; 2 -1; 2 1]  RevolutionCrossSectionUnits=m  RevolutionExtent=Full  RevolutionAngle=180  RevolutionAngleUnits=deg  BlockFunction=simmechanics.library.body_elements.solid
  F : PMIOPort  Port=1  Side=Left
  connections:
  Solid/RConn1 -- ReferenceFrame/RConn1 -- F/RConn1

== system AssemControl/Assem2_1_RIGID/straf3_dolg11_7_RIGID ==
  ReferenceFrame : sm_lib/Frames and  Transforms/Reference  Frame  BlockFunction=simmechanics.library.frames_transforms.reference_frame
  Solid : sm_lib/Body Elements/Solid  InertiaType=Custom  Mass=0.000114876  MassUnits=kg  CenterOfMass=[-1.42702 -0.0032510100000000004 0.00051650799999999994]  CenterOfMassUnits=mm  MomentsOfInertia=[0.00026421799999999998 0.0019891899999999996 0.0019891700000000002]  MomentsOfInertiaUnits=kg*mm^2  ProductsOfInertia=[-1.31544e-07 -5.9438499999999999e-07 -2.3482500000000001e-07]  ProductsOfInertiaUnits=kg*mm^2  DensityBased=on  Density=1000  DensityUnits=kg/(m^3)  GraphicType=FromGeometry  MarkerShape=Sphere  MarkerSize=10  MarkerSizeUnits=m  GraphicVisPropType=SimpleVisualProperties  GraphicDiffuseColor=[0.792157 0.819608 0.933333]  GraphicSpecularColor=[0.5 0.5 0.5 1.0]  GraphicAmbientColor=[0.15 0.15 0.15 1.0]  GraphicEmissiveColor=[0.0 0.0 0.0 1.0]  GraphicShininess=75  GraphicOpacity=1  GeometryShape=FromFile  RectangleSize=[1 1]  RectangleSizeUnits=m  BrickDimensions=[1 1 1]  BrickDimensionUnits=m  CylinderRadius=1  CylinderRadiusUnits=m  CylinderLength=1  CylinderLengthUnits=m  SphereRadius=1  SphereRadiusUnits=m  EllipsoidRadii=[1 1 1]  EllipsoidRadiiUnits=m  ExtrusionCrossSection=[1 1; -1 1; -1 -1; 1 -1]  ExtrusionCrossSectionUnits=m  ExtrusionLength=1  ExtrusionLengthUnits=m  PolygonNumSides=3  PolygonOuterRadius=1  PolygonOuterRadiusUnits=m  ExtGeomFileName=straf3_dolg11_Default_sldprt.STL  ExtGeomFileUnits=mm  RevolutionCrossSection=[1 1; 1 -1; 2 -1; 2 1]  RevolutionCrossSectionUnits=m  RevolutionExtent=Full  RevolutionAngle=180  RevolutionAngleUnits=deg  BlockFunction=simmechanics.library.body_elements.solid
  F : PMIOPort  Port=1  Side=Left
  connections:
  Solid/RConn1 -- ReferenceFrame/RConn1 -- F/RConn1

== system AssemControl/Assem2_1_RIGID/straf3_dolg11_8_RIGID ==
  ReferenceFrame : sm_lib/Frames and  Transforms/Reference  Frame  BlockFunction=simmechanics.library.frames_transforms.reference_frame
  Solid : sm_lib/Body Elements/Solid  InertiaType=Custom  Mass=0.000114876  MassUnits=kg  CenterOfMass=[-1.42702 -0.0032510100000000004 0.00051650799999999994]  CenterOfMassUnits=mm  MomentsOfInertia=[0.00026421799999999998 0.0019891899999999996 0.0019891700000000002]  MomentsOfInertiaUnits=kg*mm^2  ProductsOfInertia=[-1.31544e-07 -5.9438499999999999e-07 -2.3482500000000001e-07]  ProductsOfInertiaUnits=kg*mm^2  DensityBased=on  Density=1000  DensityUnits=kg/(m^3)  GraphicType=FromGeometry  MarkerShape=Sphere  MarkerSize=10  MarkerSizeUnits=m  GraphicVisPropType=SimpleVisualProperties  GraphicDiffuseColor=[0.792157 0.819608 0.933333]  GraphicSpecularColor=[0.5 0.5 0.5 1.0]  GraphicAmbientColor=[0.15 0.15 0.15 1.0]  GraphicEmissiveColor=[0.0 0.0 0.0 1.0]  GraphicShininess=75  GraphicOpacity=1  GeometryShape=FromFile  RectangleSize=[1 1]  RectangleSizeUnits=m  BrickDimensions=[1 1 1]  BrickDimensionUnits=m  CylinderRadius=1  CylinderRadiusUnits=m  CylinderLength=1  CylinderLengthUnits=m  SphereRadius=1  SphereRadiusUnits=m  EllipsoidRadii=[1 1 1]  EllipsoidRadiiUnits=m  ExtrusionCrossSection=[1 1; -1 1; -1 -1; 1 -1]  ExtrusionCrossSectionUnits=m  ExtrusionLength=1  ExtrusionLengthUnits=m  PolygonNumSides=3  PolygonOuterRadius=1  PolygonOuterRadiusUnits=m  ExtGeomFileName=straf3_dolg11_Default_sldprt.STL  ExtGeomFileUnits=mm  RevolutionCrossSection=[1 1; 1 -1; 2 -1; 2 1]  RevolutionCrossSectionUnits=m  RevolutionExtent=Full  RevolutionAngle=180  RevolutionAngleUnits=deg  BlockFunction=simmechanics.library.body_elements.solid
  F : PMIOPort  Port=1  Side=Left
  connections:
  Solid/RConn1 -- ReferenceFrame/RConn1 -- F/RConn1

== system AssemControl/Assem3_1_RIGID/Part2_1_RIGID ==
  ReferenceFrame : sm_lib/Frames and  Transforms/Reference  Frame  BlockFunction=simmechanics.library.frames_transforms.reference_frame
  Solid : sm_lib/Body Elements/Solid  InertiaType=Custom  Mass=0.021492799999999999  MassUnits=kg  CenterOfMass=[0 75 0]  CenterOfMassUnits=mm  MomentsOfInertia=[51.245700000000006 1.1927300000000001 52.3489]  MomentsOfInertiaUnits=kg*mm^2  ProductsOfInertia=[0 0 0]  ProductsOfInertiaUnits=kg*mm^2  DensityBased=on  Density=1000  DensityUnits=kg/(m^3)  GraphicType=FromGeometry  MarkerShape=Sphere  MarkerSize=10  MarkerSizeUnits=m  GraphicVisPropType=SimpleVisualProperties  GraphicDiffuseColor=[0.792157 0.819608 0.933333]  GraphicSpecularColor=[0.5 0.5 0.5 1.0]  GraphicAmbientColor=[0.15 0.15 0.15 1.0]  GraphicEmissiveColor=[0.0 0.0 0.0 1.0]  GraphicShininess=75  GraphicOpacity=1  GeometryShape=FromFile  RectangleSize=[1 1]  RectangleSizeUnits=m  BrickDimensions=[1 1 1]  BrickDimensionUnits=m  CylinderRadius=1  CylinderRadiusUnits=m  CylinderLength=1  CylinderLengthUnits=m  SphereRadius=1  SphereRadiusUnits=m  EllipsoidRadii=[1 1 1]  EllipsoidRadiiUnits=m  ExtrusionCrossSection=[1 1; -1 1; -1 -1; 1 -1]  ExtrusionCrossSectionUnits=m  ExtrusionLength=1  ExtrusionLengthUnits=m  PolygonNumSides=3  PolygonOuterRadius=1  PolygonOuterRadiusUnits=m  ExtGeomFileName=Part2_Default_sldprt.STL  ExtGeomFileUnits=mm  RevolutionCrossSection=[1 1; 1 -1; 2 -1; 2 1]  RevolutionCrossSectionUnits=m  RevolutionExtent=Full  RevolutionAngle=180  RevolutionAngleUnits=deg  BlockFunction=simmechanics.library.body_elements.solid
  F : PMIOPort  Port=1  Side=Left
  connections:
  Solid/RConn1 -- ReferenceFrame/RConn1 -- F/RConn1

== system AssemControl/Assem3_1_RIGID/Part2_2_RIGID ==
  ReferenceFrame : sm_lib/Frames and  Transforms/Reference  Frame  BlockFunction=simmechanics.library.frames_transforms.reference_frame
  Solid : sm_lib/Body Elements/Solid  InertiaType=Custom  Mass=0.021492799999999999  MassUnits=kg  CenterOfMass=[0 75 0]  CenterOfMassUnits=mm  MomentsOfInertia=[51.245700000000006 1.1927300000000001 52.3489]  MomentsOfInertiaUnits=kg*mm^2  ProductsOfInertia=[0 0 0]  ProductsOfInertiaUnits=kg*mm^2  DensityBased=on  Density=1000  DensityUnits=kg/(m^3)  GraphicType=FromGeometry  MarkerShape=Sphere  MarkerSize=10  MarkerSizeUnits=m  GraphicVisPropType=SimpleVisualProperties  GraphicDiffuseColor=[0.792157 0.819608 0.933333]  GraphicSpecularColor=[0.5 0.5 0.5 1.0]  GraphicAmbientColor=[0.15 0.15 0.15 1.0]  GraphicEmissiveColor=[0.0 0.0 0.0 1.0]  GraphicShininess=75  GraphicOpacity=1  GeometryShape=FromFile  RectangleSize=[1 1]  RectangleSizeUnits=m  BrickDimensions=[1 1 1]  BrickDimensionUnits=m  CylinderRadius=1  CylinderRadiusUnits=m  CylinderLength=1  CylinderLengthUnits=m  SphereRadius=1  SphereRadiusUnits=m  EllipsoidRadii=[1 1 1]  EllipsoidRadiiUnits=m  ExtrusionCrossSection=[1 1; -1 1; -1 -1; 1 -1]  ExtrusionCrossSectionUnits=m  ExtrusionLength=1  ExtrusionLengthUnits=m  PolygonNumSides=3  PolygonOuterRadius=1  PolygonOuterRadiusUnits=m  ExtGeomFileName=Part2_Default_sldprt.STL  ExtGeomFileUnits=mm  RevolutionCrossSection=[1 1; 1 -1; 2 -1; 2 1]  RevolutionCrossSectionUnits=m  RevolutionExtent=Full  RevolutionAngle=180  RevolutionAngleUnits=deg  BlockFunction=simmechanics.library.body_elements.solid
  F : PMIOPort  Port=1  Side=Left
  connections:
  Solid/RConn1 -- ReferenceFrame/RConn1 -- F/RConn1

== system AssemControl/Assem4_1_RIGID/Motor3_1_RIGID ==
  ReferenceFrame : sm_lib/Frames and  Transforms/Reference  Frame  BlockFunction=simmechanics.library.frames_transforms.reference_frame
  Solid : sm_lib/Body Elements/Solid  InertiaType=Custom  Mass=0.029311899999999998  MassUnits=kg  CenterOfMass=[0 -22.821300000000001 -9.8650699999999993]  CenterOfMassUnits=mm  MomentsOfInertia=[7.2099700000000002 5.1344899999999996 4.0333199999999998]  MomentsOfInertiaUnits=kg*mm^2  ProductsOfInertia=[0.19122700000000001 -4.5875100000000004e-09 0]  ProductsOfInertiaUnits=kg*mm^2  DensityBased=on  Density=1000  DensityUnits=kg/(m^3)  GraphicType=FromGeometry  MarkerShape=Sphere  MarkerSize=10  MarkerSizeUnits=m  GraphicVisPropType=SimpleVisualProperties  GraphicDiffuseColor=[0.25098 0.25098 0.25098]  GraphicSpecularColor=[0.5 0.5 0.5 1.0]  GraphicAmbientColor=[0.15 0.15 0.15 1.0]  GraphicEmissiveColor=[0.0 0.0 0.0 1.0]  GraphicShininess=75  GraphicOpacity=1  GeometryShape=FromFile  RectangleSize=[1 1]  RectangleSizeUnits=m  BrickDimensions=[1 1 1]  BrickDimensionUnits=m  CylinderRadius=1  CylinderRadiusUnits=m  CylinderLength=1  CylinderLengthUnits=m  SphereRadius=1  SphereRadiusUnits=m  EllipsoidRadii=[1 1 1]  EllipsoidRadiiUnits=m  ExtrusionCrossSection=[1 1; -1 1; -1 -1; 1 -1]  ExtrusionCrossSectionUnits=m  ExtrusionLength=1  ExtrusionLengthUnits=m  PolygonNumSides=3  PolygonOuterRadius=1  PolygonOuterRadiusUnits=m  ExtGeomFileName=Motor3_Default_sldprt.STL  ExtGeomFileUnits=mm  RevolutionCrossSection=[1 1; 1 -1; 2 -1; 2 1]  RevolutionCrossSectionUnits=m  RevolutionExtent=Full  RevolutionAngle=180  RevolutionAngleUnits=deg  BlockFunction=simmechanics.library.body_elements.solid
  F : PMIOPort  Port=1  Side=Left
  connections:
  Solid/RConn1 -- ReferenceFrame/RConn1 -- F/RConn1

== system AssemControl/Assem4_1_RIGID/Motor3_2_RIGID ==
  ReferenceFrame : sm_lib/Frames and  Transforms/Reference  Frame  BlockFunction=simmechanics.library.frames_transforms.reference_frame
  Solid : sm_lib/Body Elements/Solid  InertiaType=Custom  Mass=0.029311899999999998  MassUnits=kg  CenterOfMass=[0 -22.821300000000001 -9.8650699999999993]  CenterOfMassUnits=mm  MomentsOfInertia=[7.2099700000000002 5.1344899999999996 4.0333199999999998]  MomentsOfInertiaUnits=kg*mm^2  ProductsOfInertia=[0.19122700000000001 -4.5875100000000004e-09 0]  ProductsOfInertiaUnits=kg*mm^2  DensityBased=on  Density=1000  DensityUnits=kg/(m^3)  GraphicType=FromGeometry  MarkerShape=Sphere  MarkerSize=10  MarkerSizeUnits=m  GraphicVisPropType=SimpleVisualProperties  GraphicDiffuseColor=[0.25098 0.25098 0.25098]  GraphicSpecularColor=[0.5 0.5 0.5 1.0]  GraphicAmbientColor=[0.15 0.15 0.15 1.0]  GraphicEmissiveColor=[0.0 0.0 0.0 1.0]  GraphicShininess=75  GraphicOpacity=1  GeometryShape=FromFile  RectangleSize=[1 1]  RectangleSizeUnits=m  BrickDimensions=[1 1 1]  BrickDimensionUnits=m  CylinderRadius=1  CylinderRadiusUnits=m  CylinderLength=1  CylinderLengthUnits=m  SphereRadius=1  SphereRadiusUnits=m  EllipsoidRadii=[1 1 1]  EllipsoidRadiiUnits=m  ExtrusionCrossSection=[1 1; -1 1; -1 -1; 1 -1]  ExtrusionCrossSectionUnits=m  ExtrusionLength=1  ExtrusionLengthUnits=m  PolygonNumSides=3  PolygonOuterRadius=1  PolygonOuterRadiusUnits=m  ExtGeomFileName=Motor3_Default_sldprt.STL  ExtGeomFileUnits=mm  RevolutionCrossSection=[1 1; 1 -1; 2 -1; 2 1]  RevolutionCrossSectionUnits=m  RevolutionExtent=Full  RevolutionAngle=180  RevolutionAngleUnits=deg  BlockFunction=simmechanics.library.body_elements.solid
  F : PMIOPort  Port=1  Side=Left
  connections:
  Solid/RConn1 -- ReferenceFrame/RConn1 -- F/RConn1
